simulink model "SchemaROV"  (R2020a)
settings: Solver=FixedStepAuto  StartTime=0.0  StopTime=inf  FixedStep=0.00001  RelTol=1e-3
libraries: xpcutilitieslib x2, xpcrtudplib x2
settings Model: Creator=stenl  LastModifiedBy=stenl

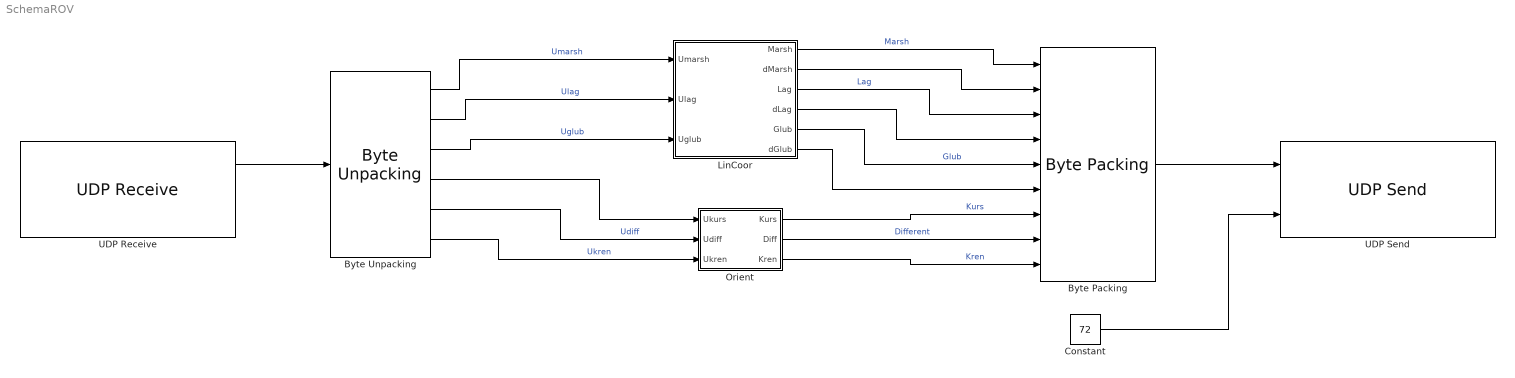
== system SchemaROV ==
  "Byte Packing " : xpcutilitieslib/Byte Packing   MaskPackedDataType=uint8  MaskUnpackedDataTypes={'double', 'double', 'double', 'double', 'double', 'double', 'double', 'double', 'double'}  MaskAlignment=1
  "Byte Unpacking " : xpcutilitieslib/Byte Unpacking   MaskUnpackedDataTypes={'double', 'double', 'double', 'double', 'double', 'double'}  MaskUnpackedDataSizes={[1], [1], [1], [1], [1], [1]}  MaskAlignment=1
      settings: SourceProductBaseCode=XP
  Constant : Constant  Value=72
  LinCoor : Subsystem
  Orient : Subsystem
  UDP Receive : xpcrtudplib/UDP Receive  ipAddressVal=Use host-target connection  localPort=13042  rcvWidth=48  rcvFmAny=on  fmAddress=0.0.0.0  rcvMulticast=off  multicastAddress={}  maxUDPQueue=8  sampleTime=0.01
  UDP Send : xpcrtudplib/UDP Send  ipAddressVal=Use host-target connection  localPort=13043  toAddress=127.0.0.1  toPort=13044  sampleTime=0.01
      settings: SourceProductBaseCode=XP
  wires:
  UDP Receive/1 -> "Byte Unpacking "/1
  "Byte Packing "/1 -> UDP Send/1
  Constant/1 -> UDP Send/2
  "Byte Unpacking "/1 -> LinCoor/1(Umarsh)  "Umarsh"
  "Byte Unpacking "/2 -> LinCoor/2(Ulag)  "Ulag"
  "Byte Unpacking "/3 -> LinCoor/3(Uglub)  "Uglub"
  "Byte Unpacking "/5 -> Orient/2(Udiff)  "Udiff"
  "Byte Unpacking "/6 -> Orient/3(Ukren)  "Ukren"
  "Byte Unpacking "/4 -> Orient/1(Ukurs)
  LinCoor/1(Marsh) -> "Byte Packing "/1  "Marsh"
  LinCoor/2(dMarsh) -> "Byte Packing "/2
  LinCoor/3(Lag) -> "Byte Packing "/3  "Lag"
  LinCoor/4(dLag) -> "Byte Packing "/4
  LinCoor/5(Glub) -> "Byte Packing "/5  "Glub"
  LinCoor/6(dGlub) -> "Byte Packing "/6
  Orient/1(Kurs) -> "Byte Packing "/7  "Kurs"
  Orient/2(Diff) -> "Byte Packing "/8  "Different"
  Orient/3(Kren) -> "Byte Packing "/9  "Kren"

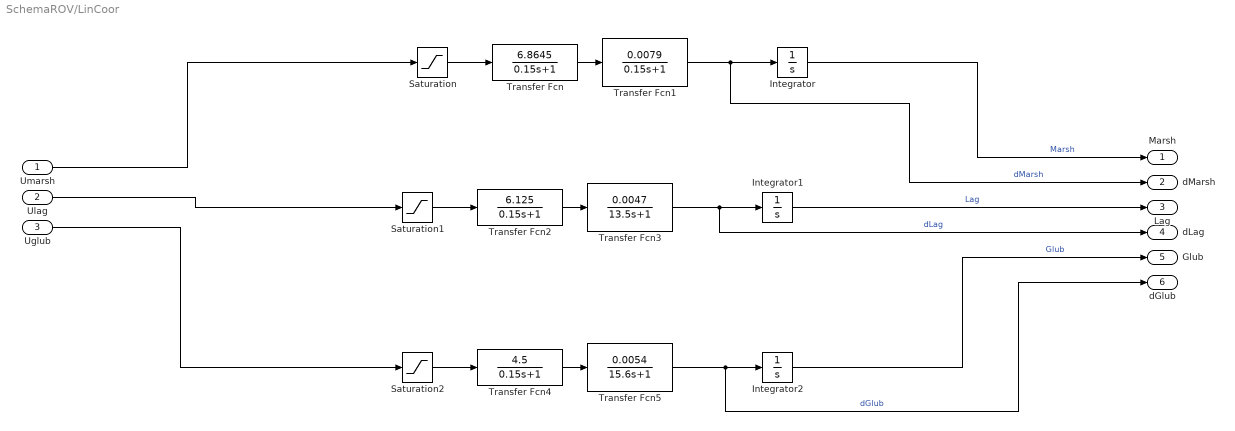
== system SchemaROV/LinCoor ==
  Umarsh : Inport
  Ulag : Inport  Port=2
  Uglub : Inport  Port=3
  Integrator : Integrator
  Integrator1 : Integrator
  Integrator2 : Integrator
  Saturation : Saturate  UpperLimit=500  LowerLimit=-500
  Saturation1 : Saturate  UpperLimit=500  LowerLimit=-500
  Saturation2 : Saturate  UpperLimit=500  LowerLimit=-500
  Transfer Fcn : TransferFcn  Numerator=[6.8645]  Denominator=[0.15 1]
  Transfer Fcn1 : TransferFcn  Numerator=[0.0079]  Denominator=[0.15 1]
  Transfer Fcn2 : TransferFcn  Numerator=[6.125]  Denominator=[0.15 1]
  Transfer Fcn3 : TransferFcn  Numerator=[0.0047]  Denominator=[13.5 1]
  Transfer Fcn4 : TransferFcn  Numerator=[4.5]  Denominator=[0.15 1]
  Transfer Fcn5 : TransferFcn  Numerator=[0.0054]  Denominator=[15.6 1]
  Marsh : Outport
  dMarsh : Outport  Port=2
  Lag : Outport  Port=3
  dLag : Outport  Port=4
  Glub : Outport  Port=5
  dGlub : Outport  Port=6
  wires:
  Transfer Fcn5/1 -> dGlub/1, Integrator2/1  "dGlub"
  Transfer Fcn4/1 -> Transfer Fcn5/1
  Transfer Fcn/1 -> Transfer Fcn1/1
  Transfer Fcn2/1 -> Transfer Fcn3/1
  Saturation2/1 -> Transfer Fcn4/1
  Transfer Fcn1/1 -> dMarsh/1, Integrator/1  "dMarsh"
  Transfer Fcn3/1 -> dLag/1, Integrator1/1  "dLag"
  Saturation/1 -> Transfer Fcn/1
  Saturation1/1 -> Transfer Fcn2/1
  Integrator2/1 -> Glub/1  "Glub"
  Integrator/1 -> Marsh/1  "Marsh"
  Integrator1/1 -> Lag/1  "Lag"
  Uglub/1 -> Saturation2/1
  Ulag/1 -> Saturation1/1
  Umarsh/1 -> Saturation/1

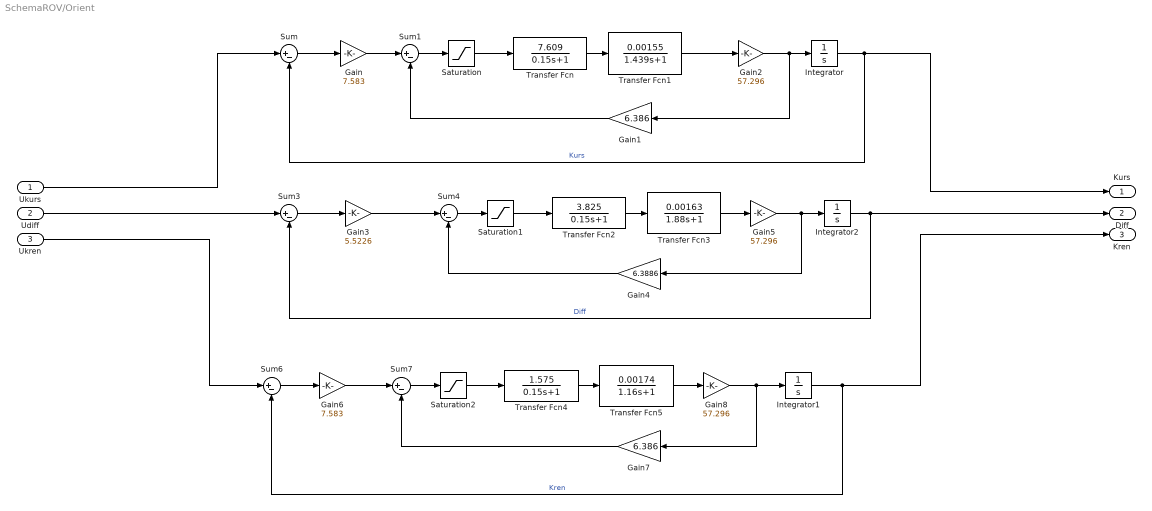
== system SchemaROV/Orient ==
  Ukurs : Inport
  Udiff : Inport  Port=2
  Ukren : Inport  Port=3
  Gain : Gain  Gain=7.583
  Gain1 : Gain  Gain=6.386
  Gain2 : Gain  Gain=57.296
  Gain3 : Gain  Gain=5.5226
  Gain4 : Gain  Gain=6.3886
  Gain5 : Gain  Gain=57.296
  Gain6 : Gain  Gain=7.583
  Gain7 : Gain  Gain=6.386
  Gain8 : Gain  Gain=57.296
  Integrator : Integrator
  Integrator1 : Integrator
  Integrator2 : Integrator
  Saturation : Saturate  UpperLimit=500  LowerLimit=-500
  Saturation1 : Saturate  UpperLimit=500  LowerLimit=-500
  Saturation2 : Saturate  UpperLimit=500  LowerLimit=-500
  Sum{,1,3..4,6..7} (6 alike) : Sum  Inputs=|+-
  Transfer Fcn : TransferFcn  Numerator=[7.609]  Denominator=[0.15 1]
  Transfer Fcn1 : TransferFcn  Numerator=[0.00155]  Denominator=[1.439 1]
  Transfer Fcn2 : TransferFcn  Numerator=[3.825]  Denominator=[0.15 1]
  Transfer Fcn3 : TransferFcn  Numerator=[0.00163]  Denominator=[1.88 1]
  Transfer Fcn4 : TransferFcn  Numerator=[1.575]  Denominator=[0.15 1]
  Transfer Fcn5 : TransferFcn  Numerator=[0.00174]  Denominator=[1.16 1]
  Kurs : Outport
  Diff : Outport  Port=2
  Kren : Outport  Port=3
  wires:
  Gain1/1 -> Sum1/2
  Gain3/1 -> Sum4/1
  Transfer Fcn4/1 -> Transfer Fcn5/1
  Gain8/1 -> Gain7/1, Integrator1/1
  Saturation1/1 -> Transfer Fcn2/1
  Transfer Fcn3/1 -> Gain5/1
  Integrator/1 -> Sum/2, Kurs/1  "Kurs"
  Sum7/1 -> Saturation2/1
  Gain5/1 -> Gain4/1, Integrator2/1
  Sum1/1 -> Saturation/1
  Integrator2/1 -> Diff/1, Sum3/2  "Diff"
  Gain6/1 -> Sum7/1
  Sum/1 -> Gain/1
  Gain2/1 -> Gain1/1, Integrator/1
  Transfer Fcn1/1 -> Gain2/1
  Saturation2/1 -> Transfer Fcn4/1
  Gain7/1 -> Sum7/2
  Sum3/1 -> Gain3/1
  Sum4/1 -> Saturation1/1
  Transfer Fcn2/1 -> Transfer Fcn3/1
  Transfer Fcn/1 -> Transfer Fcn1/1
  Gain4/1 -> Sum4/2
  Integrator1/1 -> Kren/1, Sum6/2  "Kren"
  Udiff/1 -> Sum3/1
  Gain/1 -> Sum1/1
  Ukren/1 -> Sum6/1
  Saturation/1 -> Transfer Fcn/1
  Sum6/1 -> Gain6/1
  Ukurs/1 -> Sum/1
  Transfer Fcn5/1 -> Gain8/1
